simulink model "SYS5_3"  (R2021b)
settings: Solver=FixedStepAuto  StartTime=0.0  StopTime=0.1  FixedStep=0.001  RelTol=1e-3
values from neighbouring files (symbols this model uses):
  Jn = 2*Jd    (= 0.000334)    [main.m]
  K = place(A,B,p)    [main.m]
  Kd = place(Sysd.a,Sysd.b,pd)    [main.m]
  Kdnorm1 = 1/yduk(3)    [main.m]
  km = Mn/In    (= 0.228971962617)    [main.m]
  ku = 20    [main.m]
  La = 10^-3 * 58    (= 0.058)    [main.m]
  R = 8.5    [main.m]
  Sysd = c2d(sys,Ts, 'zoh')    [main.m]
settings Model: Creator=Admin  LastModifiedBy=vkad
settings SolverCC: AlgebraicLoopSolver=TrustRegion
settings DebuggingCC: SFMachineParentedDataDiag=warning

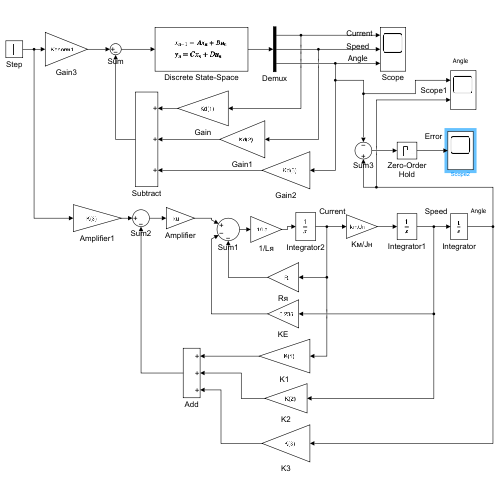
[thumbnail: Simulink's stored preview of the top-level diagram]
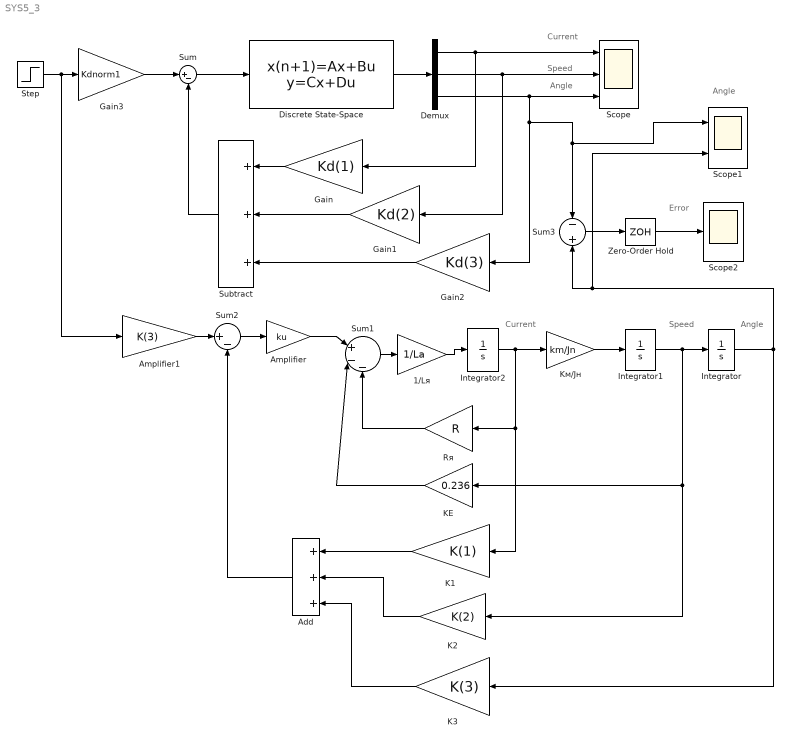
== system SYS5_3 ==
  note: Error
  note: Angle
  note: Speed
  note: Current
  note: Angle
  note: Speed
  note: Current
  note: Angle
  1/Lя : Gain  Gain=1/La
  Add : Sum  Inputs=+++
  Amplifier : Gain  Gain=ku
  Amplifier1 : Gain  Gain=K(3)
  Demux : Demux  Outputs=3
  Discrete State-Space : DiscreteStateSpace  A=Sysd.a  B=Sysd.b  C=Sysd.c  D=Sysd.d  SampleTime=0.001
  Gain : Gain  Gain=Kd(1)
  Gain1 : Gain  Gain=Kd(2)
  Gain2 : Gain  Gain=Kd(3)
  Gain3 : Gain  Gain=Kdnorm1
  Integrator : Integrator
  Integrator1 : Integrator
  Integrator2 : Integrator
  K1 : Gain  Gain=K(1)
  K2 : Gain  Gain=K(2)
  K3 : Gain  Gain=K(3)
  KE : Gain  Gain=0.236
  Kм/Jн : Gain  Gain=km/Jn
  Rя : Gain  Gain=R
  Scope : Scope  NumInputPorts=3
  Scope1 : Scope  NumInputPorts=2
  Scope2 : Scope
  Step : Step  Time=0  SampleTime=0
  Subtract : Sum  Inputs=+++
  Sum : Sum  Inputs=|+-
  Sum1 : Sum  Inputs=|+--
  Sum2 : Sum  Inputs=|+-
  Sum3 : Sum  Inputs=-+
  Zero-Order Hold : ZeroOrderHold  SampleTime=0.001
  wires:
  Discrete State-Space/1 -> Demux/1
  Demux/1 -> Gain/1, Scope/1
  Demux/3 -> Gain2/1, Scope1/1, Sum3/1, Scope/3
  Demux/2 -> Gain1/1, Scope/2
  Sum/1 -> Discrete State-Space/1
  Step/1 -> Amplifier1/1, Gain3/1
  Gain2/1 -> Subtract/3
  Gain1/1 -> Subtract/2
  Gain/1 -> Subtract/1
  Subtract/1 -> Sum/2
  Gain3/1 -> Sum/1
  Amplifier/1 -> Sum1/1
  K2/1 -> Add/2
  Integrator2/1 -> Kм/Jн/1, Rя/1, K1/1
  KE/1 -> Sum1/2
  Integrator/1 -> Sum3/2, Scope1/2, K3/1
  Sum1/1 -> 1/Lя/1
  Rя/1 -> Sum1/3
  K3/1 -> Add/3
  Kм/Jн/1 -> Integrator1/1
  Sum2/1 -> Amplifier/1
  1/Lя/1 -> Integrator2/1
  Integrator1/1 -> Integrator/1, K2/1, KE/1
  K1/1 -> Add/1
  Amplifier1/1 -> Sum2/1
  Add/1 -> Sum2/2
  Sum3/1 -> Zero-Order Hold/1
  Zero-Order Hold/1 -> Scope2/1
